simulink model "aie_testbench"  (R2022a)
settings: Solver=VariableStepAuto  StartTime=0.0  StopTime=384  RelTol=1e-3
PostLoadFcn:
  | data_in = xmcVitisRead('data/input.txt', 'cint16');
  | golden_out = xmcVitisRead('data/golden.txt', 'int32');
StopFcn:
  | % plot(data_out - double(golden_out));
  | % title('Error between Reference Output and Simulated Output');
undefined symbols (not defined in the file): S, vsva2197, xcvc1902
libraries: aieBasic x3, aieUtilities x2, dspsrcs4 x1, vmcUtilities x1
settings Model: Creator=robg  LastModifiedBy=robg
settings DataIOCC: SaveOutput=off  SignalLogging=off  DSMLogging=off  SaveTime=off  ReturnWorkspaceOutputs=off
settings DebuggingCC: UnconnectedInputMsg=warning  UnconnectedOutputMsg=warning  UnconnectedLineMsg=warning
settings RTWCC: DLArmComputeVersion=19.05

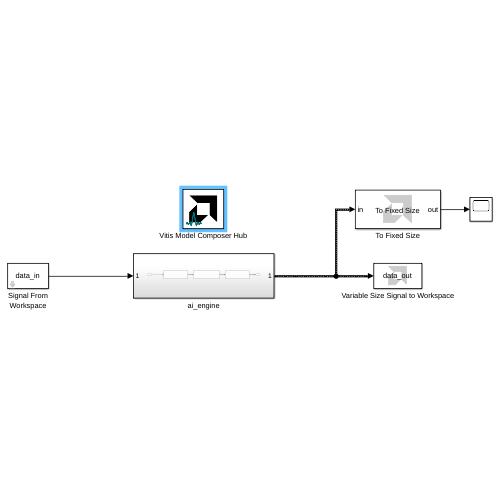
[thumbnail: Simulink's stored preview of the top-level diagram]
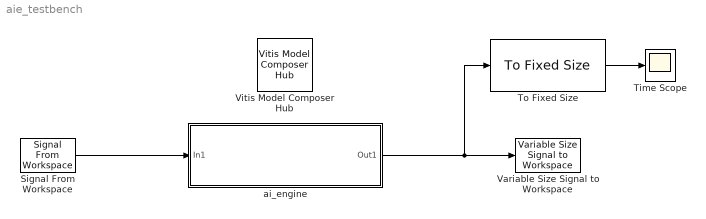
== system aie_testbench ==
  Signal From Workspace : dspsrcs4/Signal From Workspace  X=data_in  Ts=1  nsamps=128  OutputAfterFinalValue=Setting to zero  ignoreOrWarnInputAndFrameLengths=off  OutputFrames=off
  Time Scope : Scope
  To Fixed Size : aieUtilities/To Fixed Size  Mode=Stop simulation when input variable-size signal is not full  OutputSize=Inherit: Same as input  CopyMethod=Buffer samples to form output  HasStatusOutput=on
  Variable Size Signal to Workspace : aieUtilities/Variable Size Signal to Workspace  VariableNameMask=data_out
  Vitis Model Composer Hub : vmcUtilities/Vitis Model Composer Hub  Tag=genX  CodeGeneration=off  SubsystemName=ai_engine  TargetDirectory=./code  ExportType=AI Engines  IpVendor=xilinx.com  IpLibrary=hls  IpVersion=1.0  IpHWLanguage=Verilog  AieCompilerOptions={}  AieSimulatorOptions={}  CreateTestbench=off  TestbenchStackSize=10  RunRtlSim=off  RunCSim=off  RunAieSim=off  AieSimTimeout=50000  RunAieSimProfiling=off  LaunchVitisAnalyzer=off  PlotOutput=off  RunX86Sim=off  X86SimTimeout=10  GenHwImage=off  GenLibadfXo=off  PlatformType=Specify Platform  Platform=/proj/xbuilds/SWIP/2023.2_1013_0023/installs/lin64/Vitis/2023.2/base_platforms/xilinx_vck190_base_202320_1/xilinx_vck190_base_202320_1.xpfm  HwSystemType=Baremetal  HwValidationTarget=hw  ProjDevice=Versal VCK190 Evaluation Platform (xcvc1902-vsva2197-2MP-e-S)  ProjDevicePart=xcvc1902-vsva2197-2MP-e-S  AIEType=AIE  SamplePeriod=-1  ClockFrequency=200  DataPathParallelism=1  xilinxfamily=versalaicore  part=xcvc1902  speed=-2MP-e-S  package=vsva2197  directory=./netlist  testbench=off  incr_netlist=off  synthesis_tool=Vivado  clock_wrapper=Clock Enables  dbl_ovrd=According to Block Masks  dcm_input_clock_period=10  sysclk_period=10  simulink_period=1  eval_field=0  IPInfoJsonString="{\"AIESubsystem\":{\"SubsystemName\":\"ai_engine\",\"TargetDirectory\":\"./code\",\"SubsystemDir\":\"./code/ip/ai_engine\"}}"  LogFileName=/proj/xcoswmktg/robg/git/vmc_examples/Vitis_Model_Composer/Examples/AIENGINE/Export_to_Vitis/code/model_composer.log  NThreads=4
  ai_engine : Subsystem
  wires:
  To Fixed Size/1 -> Time Scope/1
  ai_engine/1(Out1) -> To Fixed Size/1, Variable Size Signal to Workspace/1
  Signal From Workspace/1 -> ai_engine/1(In1)

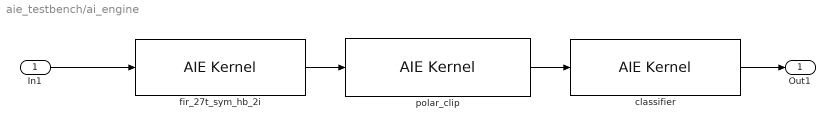
== system aie_testbench/ai_engine ==
  In1 : Inport
  classifier : aieBasic/AIE Kernel  KernelAllAttrs=s[12;12;9;9;19;14;21;23;21;23;24;21;15;17;12;24;26;26;26;27;28;9;21;23;23;23;24;25;14;19;19;29]@FunctionNameDeclFileNamePortNamesPortTypesPortSerializedTypesPortDirectionsPortWindowSizeEnablesPortWindowMarginEnablesPortBufferSizeEnablesPortBufferMarginEnablesPortSynchronicityEnablesPortSignalSizeEnablesPortBufferSizesPortBufferMarginsFunctionDeclFunctionTemplateSpecKindFunctionTemplateParamNamesFunctionTemplateParamKindsFunctionTemplateParamTypesFunctionTemplateParamValuesFunctionTemplateParamEnablesClassDeclClassTemplateSpecKindClassTemplateParamNamesClassTemplateParamKindsClassTemplateParamTypesClassTemplateParamValuesClassTemplateParamEnablesClassCtorDeclsClassCtorParamNamesClassCtorParamTypesClassCtorParamSerializedTypes[1 1]@C[32 1]@t10@classifiert19@../../aie/kernels.hC[2 1]@t5@inputt6@outputC[2 1]@t21@input_stream_cint16 *t38@adf::output_buffer< int32 > & restrictC[2 1]@t33@{P{Tinput_stream{1{t{Scint16}}}}}t40@{Q2{R{Tadf::output_buffer{1{t{Bi32}}}}}}C[2 1]@t5@inputt6@outputC[2 1]@l0@l1@C[2 1]@l0@l0@C[2 1]@l0@l1@C[2 1]@l0@l0@C[2 1]@l0@l1@C[2 1]@l0@l0@C[2 1]@nnC[2 1]@nnt91@void classifier(input_stream_cint16 * input, adf::output_buffer< int32 > & restrict output)t4@nonee[0 1]@e[0 1]@e[0 1]@e[0 1]@e[0 1]@nne[0 1]@e[0 1]@e[0 1]@e[0 1]@e[0 1]@e[0 1]@e[0 1]@e[0 1]@e[0 1]@  PortNames={'input'; 'output'}  PortSerializedTypes={'{P{Tinput_stream{1{t{Scint16}}}}}'; '{Q2{R{Tadf::output_buffer{1{t{Bi32}}}}}}'}  PortWindowSizes={0.000000000000000000e+00, 2.560000000000000000e+02}  PortWindowMargins={0.000000000000000000e+00, 0.000000000000000000e+00}  PortSynchronicities={'auto', 'sync'}  PortSignalSizes={0.000000000000000000e+00; 0.000000000000000000e+00}  FunctionTemplateSpecKind=none  FunctionTemplateParamNames={}  FunctionTemplateParamKinds={}  FunctionTemplateParamTypes={}  FunctionTemplateParamValues={}  FunctionIndex=1  FunctionTabVisible=on  FunctionTemplateParamsVisible=off  FunctionDeclTypeOptions=C[1 1]@t92@void classifier(input_stream_cint16 * input, adf::output_buffer< int32 > && restrict output)  FunctionDecl=void classifier(input_stream_cint16 * input, adf::output_buffer< int32 > && restrict output)  FunctionTemplateParams={}  FunctionTemplateParamsEnables={}  PortAttrs={ 'input', 'input', 'input_stream_cint16 *', '', '', '', ''; 'output', 'output', 'adf::output_buffer< int32 > & restrict', '256', '', 'sync', '' }  PortAttrsEnables={'off', 'off', 'off', 'off', 'off', 'off', 'off';'off', 'off', 'off', 'on', 'off', 'off', 'off'}  SampleTime=-1  KernelHeaderFile=aie/kernels.h  KernelFunction=classifier  KernelSourceFile=aie/kernels/classifiers/classify.cc  KernelSearchPaths={'./aie'}  PreProcOptions={}  blockJsonConstraints=[]
  fir_27t_sym_hb_2i : aieBasic/AIE Kernel  KernelAllAttrs=s[12;12;9;9;19;14;21;23;21;23;24;21;15;17;12;24;26;26;26;27;28;9;21;23;23;23;24;25;14;19;19;29]@FunctionNameDeclFileNamePortNamesPortTypesPortSerializedTypesPortDirectionsPortWindowSizeEnablesPortWindowMarginEnablesPortBufferSizeEnablesPortBufferMarginEnablesPortSynchronicityEnablesPortSignalSizeEnablesPortBufferSizesPortBufferMarginsFunctionDeclFunctionTemplateSpecKindFunctionTemplateParamNamesFunctionTemplateParamKindsFunctionTemplateParamTypesFunctionTemplateParamValuesFunctionTemplateParamEnablesClassDeclClassTemplateSpecKindClassTemplateParamNamesClassTemplateParamKindsClassTemplateParamTypesClassTemplateParamValuesClassTemplateParamEnablesClassCtorDeclsClassCtorParamNamesClassCtorParamTypesClassCtorParamSerializedTypes[1 1]@C[32 1]@t17@fir_27t_sym_hb_2it19@../../aie/kernels.hC[2 1]@t8@cb_inputt9@cb_outputC[2 1]@t96@adf::input_buffer< cint16, adf::extents< adf::inherited_extent >, adf::margin< 16 > > & restrictt39@adf::output_buffer< cint16 > & restrictC[2 1]@t116@{Q2{R{Tadf::input_buffer{3{t{Scint16}}{t{Tadf::extents{1{t{}adf::inherited_extent}}}}{t{Tadf::margin{1{t{}16}}}}}}}}t43@{Q2{R{Tadf::output_buffer{1{t{Scint16}}}}}}C[2 1]@t5@inputt6@outputC[2 1]@l1@l1@C[2 1]@l1@l0@C[2 1]@l1@l1@C[2 1]@l0@l0@C[2 1]@l1@l1@C[2 1]@l0@l0@C[2 1]@nnC[2 1]@t2@16nt180@void fir_27t_sym_hb_2i(adf::input_buffer< cint16, adf::extents< adf::inherited_extent >, adf::margin< 16 > > & restrict cb_input, adf::output_buffer< cint16 > & restrict cb_output)t4@nonee[0 1]@e[0 1]@e[0 1]@e[0 1]@e[0 1]@nne[0 1]@e[0 1]@e[0 1]@e[0 1]@e[0 1]@e[0 1]@e[0 1]@e[0 1]@e[0 1]@  PortNames={'cb_input'; 'cb_output'}  PortSerializedTypes={'{Q2{R{Tadf::input_buffer{3{t{Scint16}}{t{Tadf::extents{1{t{}adf::inherited_extent}}}}{t{Tadf::margin{1{t{}16}}}}}}}}'; '{Q2{R{Tadf::output_buffer{1{t{Scint16}}}}}}'}  PortWindowSizes={1.280000000000000000e+02, 2.560000000000000000e+02}  PortWindowMargins={1.600000000000000000e+01, 0.000000000000000000e+00}  PortSynchronicities={'sync', 'sync'}  PortSignalSizes={0.000000000000000000e+00; 0.000000000000000000e+00}  FunctionTemplateSpecKind=none  FunctionTemplateParamNames={}  FunctionTemplateParamKinds={}  FunctionTemplateParamTypes={}  FunctionTemplateParamValues={}  FunctionIndex=1  FunctionTabVisible=on  FunctionTemplateParamsVisible=off  FunctionDeclTypeOptions=C[1 1]@t182@void fir_27t_sym_hb_2i(adf::input_buffer< cint16, adf::extents< adf::inherited_extent >, adf::margin< 16 > > && restrict cb_input, adf::output_buffer< cint16 > && restrict cb_output)  FunctionDecl=void fir_27t_sym_hb_2i(adf::input_buffer< cint16, adf::extents< adf::inherited_extent >, adf::margin< 16 > > && restrict cb_input, adf::output_buffer< cint16 > && restrict cb_output)  FunctionTemplateParams={}  FunctionTemplateParamsEnables={}  PortAttrs={ 'input', 'cb_input', 'adf::input_buffer< cint16, adf::extents< adf::inherited_extent >, adf::margin< 16 > > & restrict', '128', '16', 'sync', ''; 'output', 'cb_output', 'adf::output_buffer< cint16 > & restrict', '256', '', 'sync', '' }  PortAttrsEnables={'off', 'off', 'off', 'on', 'off', 'off', 'off';'off', 'off', 'off', 'on', 'off', 'off', 'off'}  SampleTime=-1  KernelHeaderFile=aie/kernels.h  KernelFunction=fir_27t_sym_hb_2i  KernelSourceFile=aie/kernels/interpolators/hb27_2i.cc  KernelSearchPaths={'./aie'}  PreProcOptions={}  blockJsonConstraints=[]
  polar_clip : aieBasic/AIE Kernel  KernelAllAttrs=s[12;12;9;9;19;14;21;23;21;23;24;21;15;17;12;24;26;26;26;27;28;9;21;23;23;23;24;25;14;19;19;29]@FunctionNameDeclFileNamePortNamesPortTypesPortSerializedTypesPortDirectionsPortWindowSizeEnablesPortWindowMarginEnablesPortBufferSizeEnablesPortBufferMarginEnablesPortSynchronicityEnablesPortSignalSizeEnablesPortBufferSizesPortBufferMarginsFunctionDeclFunctionTemplateSpecKindFunctionTemplateParamNamesFunctionTemplateParamKindsFunctionTemplateParamTypesFunctionTemplateParamValuesFunctionTemplateParamEnablesClassDeclClassTemplateSpecKindClassTemplateParamNamesClassTemplateParamKindsClassTemplateParamTypesClassTemplateParamValuesClassTemplateParamEnablesClassCtorDeclsClassCtorParamNamesClassCtorParamTypesClassCtorParamSerializedTypes[1 1]@C[32 1]@t10@polar_clipt19@../../aie/kernels.hC[2 1]@t2@int3@outC[2 1]@t21@input_stream_cint16 *t22@output_stream_cint16 *C[2 1]@t33@{P{Tinput_stream{1{t{Scint16}}}}}t34@{P{Toutput_stream{1{t{Scint16}}}}}C[2 1]@t5@inputt6@outputC[2 1]@l0@l0@C[2 1]@l0@l0@C[2 1]@l0@l0@C[2 1]@l0@l0@C[2 1]@l0@l0@C[2 1]@l0@l1@C[2 1]@nnC[2 1]@nnt69@void polar_clip(input_stream_cint16 * in, output_stream_cint16 * out)t4@nonee[0 1]@e[0 1]@e[0 1]@e[0 1]@e[0 1]@nne[0 1]@e[0 1]@e[0 1]@e[0 1]@e[0 1]@e[0 1]@e[0 1]@e[0 1]@e[0 1]@  PortNames={'in'; 'out'}  PortSerializedTypes={'{P{Tinput_stream{1{t{Scint16}}}}}'; '{P{Toutput_stream{1{t{Scint16}}}}}'}  PortWindowSizes={0.000000000000000000e+00, 0.000000000000000000e+00}  PortWindowMargins={0.000000000000000000e+00, 0.000000000000000000e+00}  PortSynchronicities={'auto', 'auto'}  PortSignalSizes={0.000000000000000000e+00; 2.560000000000000000e+02}  FunctionTemplateSpecKind=none  FunctionTemplateParamNames={}  FunctionTemplateParamKinds={}  FunctionTemplateParamTypes={}  FunctionTemplateParamValues={}  FunctionIndex=1  FunctionTabVisible=on  FunctionTemplateParamsVisible=off  FunctionDeclTypeOptions=C[1 1]@t69@void polar_clip(input_stream_cint16 * in, output_stream_cint16 * out)  FunctionDecl=void polar_clip(input_stream_cint16 * in, output_stream_cint16 * out)  FunctionTemplateParams={}  FunctionTemplateParamsEnables={}  PortAttrs={ 'input', 'in', 'input_stream_cint16 *', '', '', '', ''; 'output', 'out', 'output_stream_cint16 *', '', '', '', '256' }  PortAttrsEnables={'off', 'off', 'off', 'off', 'off', 'off', 'off';'off', 'off', 'off', 'off', 'off', 'off', 'on'}  SampleTime=-1  KernelHeaderFile=aie/kernels.h  KernelFunction=polar_clip  KernelSourceFile=aie/kernels/polar_clip.cpp  KernelSearchPaths={'./aie'}  PreProcOptions={}  blockJsonConstraints=[]
  Out1 : Outport
  wires:
  polar_clip/1 -> classifier/1
  fir_27t_sym_hb_2i/1 -> polar_clip/1
  classifier/1 -> Out1/1
  In1/1 -> fir_27t_sym_hb_2i/1
